simulink model "inner_loop_simulation_old"  (R2020a)
settings: Solver=VariableStepAuto  StartTime=0.0  StopTime=10.0  RelTol=1e-3
settings Model: Creator=joelm  LastModifiedBy=aurel

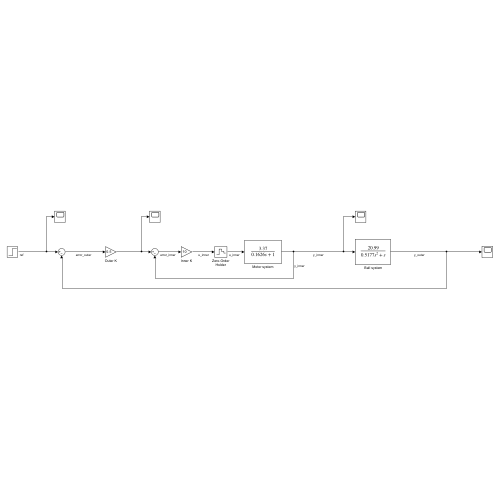
[thumbnail: Simulink's stored preview of the top-level diagram]
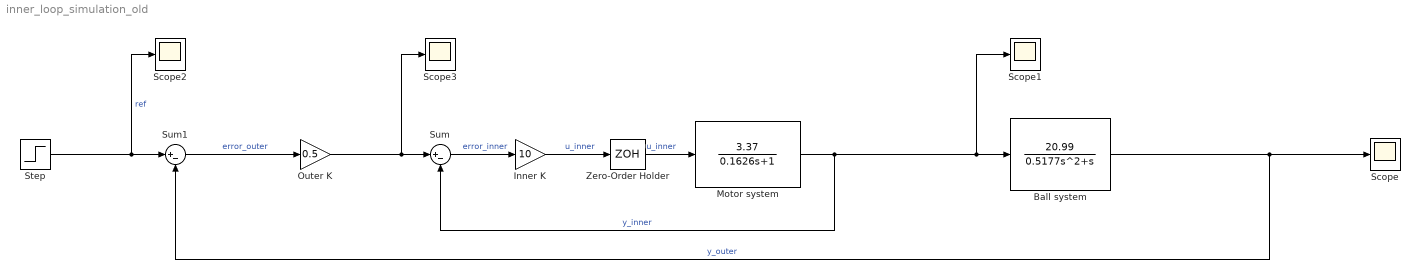
== system inner_loop_simulation_old ==
  " Ball system" : TransferFcn  Numerator=[ 20.99]  Denominator=[0.5177 1 0]
  Inner K : Gain  Gain=10
  Motor system : TransferFcn  Numerator=[0 3.37]  Denominator=[0.1626 1]
  Outer K : Gain  Gain=0.5
  Scope{,1..3} (4 alike) : Scope
  Step : Step
  Sum : Sum  Inputs=|+-
  Sum1 : Sum  Inputs=|+-
  Zero-Order Holder : ZeroOrderHold  SampleTime=0.005
  wires:
  " Ball system"/1 -> Scope/1, Sum1/2  "y_outer"
  Zero-Order Holder/1 -> Motor system/1  "u_inner"
  Motor system/1 -> Sum/2, Scope1/1, " Ball system"/1  "y_inner"
  Step/1 -> Sum1/1, Scope2/1  "ref"
  Sum1/1 -> Outer K/1  "error_outer"
  Inner K/1 -> Zero-Order Holder/1  "u_inner"
  Outer K/1 -> Sum/1, Scope3/1
  Sum/1 -> Inner K/1  "error_inner"
